simulink model "Roomba_Output_Cartesian"  (R2022b)
settings: Solver=FixedStepAuto  StartTime=0.0  StopTime=inf  FixedStep=0.02  RelTol=1e-3
undefined symbols (not defined in the file): b, offset_x, offset_y, theta_des, unicycle, X, x_des, x_f, Y, y_des, y_f
libraries: robotlib x3, dspsigops x1, simulink_extras x1
settings Model: Creator=Musta  LastModifiedBy=Musta
settings OptimizationCC: EnhancedBackFolding=on  PassReuseOutputArgsAs=Individual arguments  ZeroExternalMemoryAtStartup=off  ZeroInternalMemoryAtStartup=off  MaxStackSize=64  OptimizeBlockOrder=speed  DifferentSizesBufferReuse=on  OptimizationCustomize=off  EfficientTunableParamExpr=on
settings DebuggingCC: ParameterTunabilityLossMsg=error
settings HardwareCC: ProdBitPerPointer=32  ProdBitPerSizeT=32  ProdBitPerPtrDiffT=32  ProdLargestAtomicFloat=None  ProdIntDivRoundTo=Undefined  ProdEndianess=Unspecified  ProdWordSize=32  ProdHWDeviceType=Generic->Unspecified (assume 32-bit Generic)
settings SFSimCC: MATLABDynamicMemAlloc=off
settings RTWCC: Description=Embedded Coder  SystemTargetFile=ert.tlc  HardwareBoard=Robot Operating System (ROS)  TLCOptions="-aInlineSetEventsForThisBaseRateFcn=TLC_FALSE -aSuppressMultiTaskScheduler=TLC_FALSE  -aRateBasedStepFcn=0"  TemplateMakefile=ert_default_tmf  Toolchain=Catkin  TargetLang=C++
settings CodeAppCC: ForceParamTrailComments=on  IgnoreCustomStorageClasses=off  OperatorAnnotations=on  SimulinkDataObjDesc=on  SFDataObjDesc=on  InsertBlockDesc=on

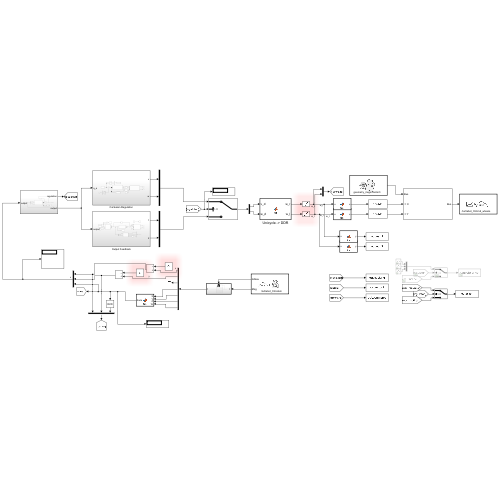
[thumbnail: Simulink's stored preview of the top-level diagram]
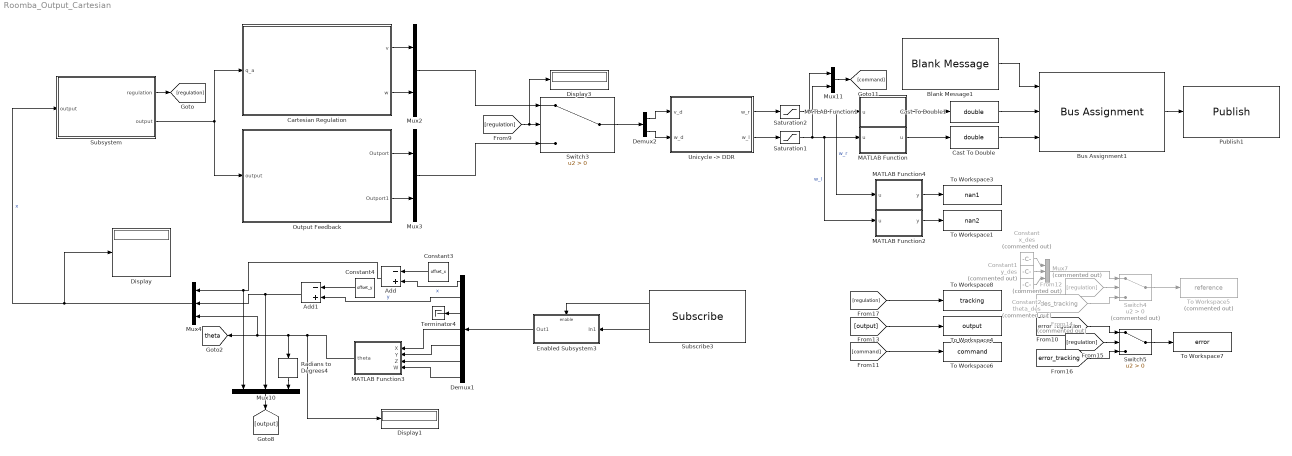
== system Roomba_Output_Cartesian ==
  Add : Sum  Inputs=-+
  Add1 : Sum  Inputs=-+
  Blank Message1 : robotlib/Blank Message  messageClass=Message  entityType=geometry_msgs/Vector3  messageType=geometry_msgs/Vector3  SampleTime=0.02  legacyBusStruct=off
      settings: LibrarySourceBlock=roslib/ROS/Blank Message
  Bus Assignment1 : BusAssignment  AssignedSignals=X,Y
  Cartesian Regulation : Subsystem
  Cast To Double : DataTypeConversion  OutDataTypeStr=double  SaturateOnIntegerOverflow=off  RndMeth=Floor
  Cast To Double1 : DataTypeConversion  OutDataTypeStr=double  SaturateOnIntegerOverflow=off  RndMeth=Floor
  Constant : Constant  Commented=on  Value=x_des
  Constant1 : Constant  Commented=on  Value=y_des
  Constant2 : Constant  Commented=on  Value=theta_des
  Constant3 : Constant  Value=offset_x
  Constant4 : Constant  Value=offset_y
  Demux1 : Demux  Outputs=7
  Demux2 : Demux  Outputs=2
  Display : Display
  Display1 : Display
  Display3 : Display
  Enabled Subsystem3 : Subsystem  TreatAsAtomicUnit=on
  From12 : From  Commented=on  GotoTag=regulation
  From14 : From  Commented=on  GotoTag=des_tracking  TagVisibility=global
  MATLAB Function : MATLAB Function  TreatAsAtomicUnit=on
  MATLAB Function1 : MATLAB Function  TreatAsAtomicUnit=on
  MATLAB Function2 : MATLAB Function  TreatAsAtomicUnit=on
  MATLAB Function3 : MATLAB Function  TreatAsAtomicUnit=on
  MATLAB Function4 : MATLAB Function  TreatAsAtomicUnit=on
  Mux10 : Mux  Inputs=3
  Mux11 : Mux  Inputs=2
  Mux2 : Mux  Inputs=2
  Mux3 : Mux  Inputs=2
  Mux4 : Mux  Inputs=3
  Mux7 : Mux  Commented=on  Inputs=3
  Output Feedback : Subsystem
  Publish1 : robotlib/Publish  topicSource=Select from ROS network  topic=/turtlebot_03/cmd_wheels  messageType=geometry_msgs/Vector3  legacyBusStruct=off  messageQueueLength=1
      settings: LibrarySourceBlock=roslib/ROS/Publish
  Radians to Degrees4 : simulink_extras/Transformations/Radians to Degrees
  Saturation1 : Saturate  UpperLimit=unicycle.omegaWheelMax  LowerLimit=unicycle.omegaWheelMin
  Saturation2 : Saturate  UpperLimit=unicycle.omegaWheelMax  LowerLimit=unicycle.omegaWheelMin
  Subscribe3 : robotlib/Subscribe  topicSource=Select from ROS network  topic=/turtlebot_03/odom  messageType=nav_msgs/Odometry  SampleTime=0.02  legacyBusStruct=off  messageQueueLength=1
      settings: LibrarySourceBlock=roslib/ROS/Subscribe
  Subsystem : Subsystem
  Switch3 : Switch  Criteria=u2 > Threshold  SaturateOnIntegerOverflow=off  InputSameDT=off
  Switch4 : Switch  Commented=on  Criteria=u2 > Threshold  SaturateOnIntegerOverflow=off  InputSameDT=off
  Switch5 : Switch  Criteria=u2 > Threshold  SaturateOnIntegerOverflow=off  InputSameDT=off
  Terminator4 : Terminator
  To Workspace1 : ToWorkspace  VariableName=nan2  SaveFormat=Structure With Time  SampleTime=-1
  To Workspace3 : ToWorkspace  VariableName=nan1  SaveFormat=Structure With Time  SampleTime=-1
  To Workspace4 : ToWorkspace  VariableName=output  SaveFormat=Structure With Time  SampleTime=-1
  To Workspace5 : ToWorkspace  Commented=on  VariableName=reference  SaveFormat=Structure With Time  SampleTime=-1
  To Workspace6 : ToWorkspace  VariableName=command  SaveFormat=Structure With Time  SampleTime=-1
  To Workspace7 : ToWorkspace  VariableName=error  SaveFormat=Structure With Time  SampleTime=-1
  To Workspace8 : ToWorkspace  VariableName=tracking  SaveFormat=Structure With Time  SampleTime=-1
  "Unicycle -> DDR" : MATLAB Function  TreatAsAtomicUnit=on
  tag scope: theta=global
  wires:
  Radians to Degrees4/1 -> Mux10/3
  "Unicycle -> DDR"/1(w_r) -> Saturation2/1
  MATLAB Function3/1(theta) -> Display1/1, Radians to Degrees4/1, Mux4/3, [theta]
  Subscribe3/2 -> Enabled Subsystem3/1(In1)
  Mux10/1 -> [output]
  Demux1/3 -> Terminator4/1
  Blank Message1/1 -> Bus Assignment1/1
  Bus Assignment1/1 -> Publish1/1
  Subscribe3/1 -> Enabled Subsystem3/Enable
  Mux11/1 -> [command]
  Enabled Subsystem3/1(Out1) -> Demux1/1
  From12/1 -> Switch4/2
  [regulation] -> To Workspace8/1
  Switch5/1 -> To Workspace7/1
  Constant1/1 -> Mux7/2
  Mux7/1 -> Switch4/1
  Demux2/2 -> "Unicycle -> DDR"/2(w_d)
  [output] -> To Workspace4/1
  [error_regulation] -> Switch5/1
  Constant/1 -> Mux7/1
  "Unicycle -> DDR"/2(w_l) -> Saturation1/1
  [regulation] -> Switch5/2
  From14/1 -> Switch4/3
  Switch4/1 -> To Workspace5/1
  Demux2/1 -> "Unicycle -> DDR"/1(v_d)
  [regulation] -> Display3/1, Switch3/2
  Mux2/1 -> Switch3/1
  [command] -> To Workspace6/1
  Switch3/1 -> Demux2/1
  [error_tracking] -> Switch5/3
  Mux3/1 -> Switch3/3
  Constant2/1 -> Mux7/3
  Mux4/1 -> Subsystem/1("output "), Display/1  "x"
  Demux1/1 -> Add/2  "x"
  Constant3/1 -> Add/1
  Constant4/1 -> Add1/1
  Demux1/2 -> Add1/2  "y"
  Add1/1 -> Mux4/2, Mux10/2
  Add/1 -> Mux4/1, Mux10/1
  Cast To Double1/1 -> Bus Assignment1/2
  Cast To Double/1 -> Bus Assignment1/3
  Output Feedback/2(Outport1) -> Mux3/2
  Output Feedback/1(Outport) -> Mux3/1
  Cartesian Regulation/1(v) -> Mux2/1
  Cartesian Regulation/2(w) -> Mux2/2
  Demux1/7 -> MATLAB Function3/4(W)
  Demux1/6 -> MATLAB Function3/3(Z)
  Demux1/4 -> MATLAB Function3/1(X)
  Demux1/5 -> MATLAB Function3/2(Y)
  Saturation1/1 -> MATLAB Function2/1(u), MATLAB Function/1("u "), Mux11/2  "w_l"
  Saturation2/1 -> MATLAB Function4/1(u), MATLAB Function1/1("u "), Mux11/1  "w_r"
  MATLAB Function/1(u) -> Cast To Double/1
  MATLAB Function2/1(y) -> To Workspace1/1
  MATLAB Function4/1(y) -> To Workspace3/1
  MATLAB Function1/1(u) -> Cast To Double1/1
  Subsystem/1(regulation) -> [regulation]
  Subsystem/2(output) -> Output Feedback/1(output), Cartesian Regulation/1(q_a)

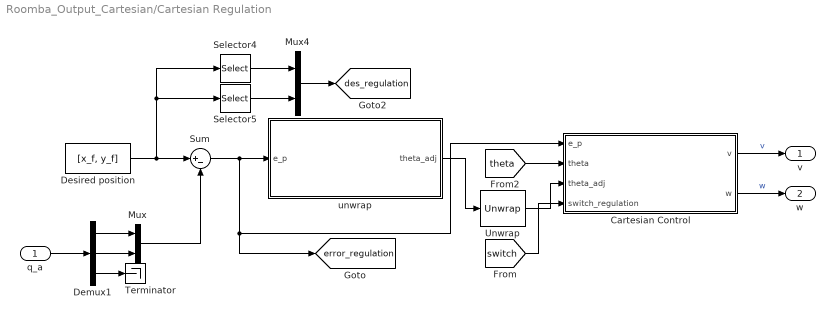
== system Roomba_Output_Cartesian/Cartesian Regulation ==
  q_a : Inport
  Cartesian Control : MATLAB Function  TreatAsAtomicUnit=on
  Demux1 : Demux  Outputs=3
  Desired position : Constant  Value=[x_f, y_f]
  Mux : Mux  Inputs=2
  Mux4 : Mux  Inputs=2
  Selector4 : Selector  InputPortWidth=2  IndexOptions=Index vector (dialog)  Indices=1  OutputSizes=1
  Selector5 : Selector  InputPortWidth=2  IndexOptions=Index vector (dialog)  Indices=2  OutputSizes=1
  Sum : Sum  Inputs=|+-
  Terminator : Terminator
  Unwrap : dspsigops/Unwrap  tol=0.99*pi  InputProcessing=Columns as channels (frame based)  running=off
  unwrap : MATLAB Function  TreatAsAtomicUnit=on
  v : Outport
  w : Outport  Port=2
  tag scope: des_regulation=global, error_regulation=global
  wires:
  Demux1/1 -> Mux/1
  Demux1/2 -> Mux/2
  q_a/1 -> Demux1/1
  unwrap/1(theta_adj) -> Unwrap/1
  Sum/1 -> [error_regulation], Cartesian Control/1(e_p), unwrap/1(e_p)
  Mux4/1 -> [des_regulation]
  Selector5/1 -> Mux4/2
  [theta] -> Cartesian Control/2(theta)
  Desired position/1 -> Selector4/1, Selector5/1, Sum/1
  Selector4/1 -> Mux4/1
  Unwrap/1 -> Cartesian Control/3(theta_adj)
  Mux/1 -> Sum/2
  Demux1/3 -> Terminator/1
  Cartesian Control/1(v) -> v/1  "v"
  Cartesian Control/2(w) -> w/1  "w"
  [switch] -> Cartesian Control/4(switch_regulation)

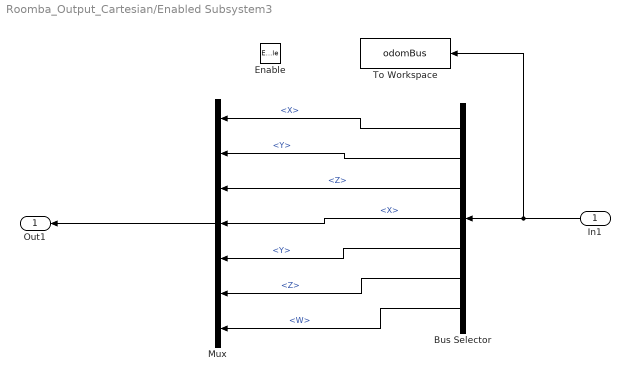
== system Roomba_Output_Cartesian/Enabled Subsystem3 ==
  In1 : Inport
  Enable : EnablePort
  Bus Selector : BusSelector  OutputSignals=Pose.Pose.Position.X,Pose.Pose.Position.Y,Pose.Pose.Position.Z,Pose.Pose.Orientation.X,Pose.Pose.Orientation.Y,Pose.Pose.Orientation.Z,Pose.Pose.Orientation.W
  Mux : Mux  Inputs=7
  To Workspace : ToWorkspace  VariableName=odomBus  SaveFormat=Timeseries  SampleTime=-1
  Out1 : Outport
  wires:
  Mux/1 -> Out1/1
  Bus Selector/1 -> Mux/1  "<X>"
  Bus Selector/2 -> Mux/2  "<Y>"
  In1/1 -> To Workspace/1, Bus Selector/1
  Bus Selector/3 -> Mux/3  "<Z>"
  Bus Selector/4 -> Mux/4  "<X>"
  Bus Selector/5 -> Mux/5  "<Y>"
  Bus Selector/6 -> Mux/6  "<Z>"
  Bus Selector/7 -> Mux/7  "<W>"

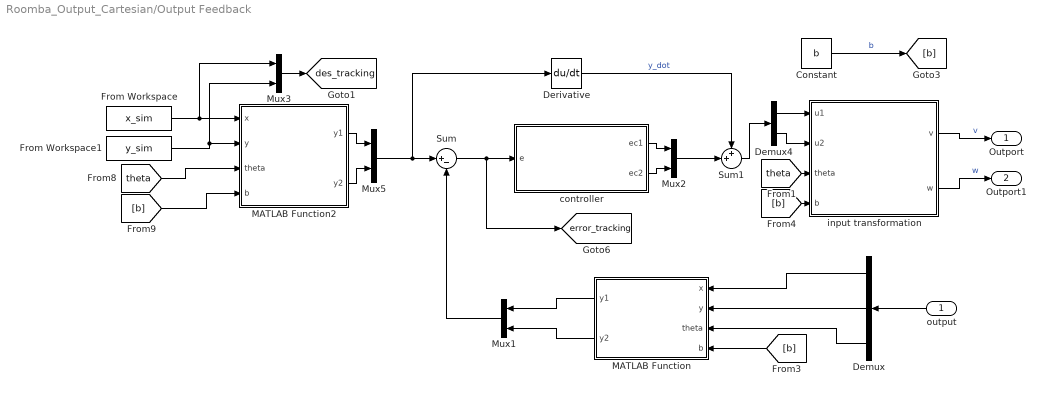
== system Roomba_Output_Cartesian/Output Feedback ==
  output : Inport
  Constant : Constant  Value=b
  Demux : Demux  Outputs=3
  Demux4 : Demux  Outputs=2
  Derivative : Derivative
  From Workspace : FromWorkspace  VariableName=x_sim
  From Workspace1 : FromWorkspace  VariableName=y_sim
  MATLAB Function : MATLAB Function  TreatAsAtomicUnit=on
  MATLAB Function2 : MATLAB Function  TreatAsAtomicUnit=on
  Mux{1..3,5} (4 alike) : Mux  Inputs=2
  Sum : Sum  Inputs=|+-
  Sum1 : Sum  Inputs=++|
  controller : MATLAB Function  TreatAsAtomicUnit=on
  input transformation : MATLAB Function  TreatAsAtomicUnit=on
  Outport : Outport
  Outport1 : Outport  Port=2
  tag scope: des_tracking=global, error_tracking=global
  wires:
  controller/1(ec1) -> Mux2/1
  Mux5/1 -> Derivative/1, Sum/1
  MATLAB Function2/2(y2) -> Mux5/2
  Mux3/1 -> [des_tracking]
  [b] -> MATLAB Function2/4(b)
  Derivative/1 -> Sum1/1  "y_dot"
  [b] -> input transformation/4(b)
  Demux4/2 -> input transformation/2(u2)
  Demux4/1 -> input transformation/1(u1)
  [theta] -> MATLAB Function2/3(theta)
  Sum/1 -> [error_tracking], controller/1(e)
  From Workspace1/1 -> Mux3/2, MATLAB Function2/2(y)
  Mux1/1 -> Sum/2
  MATLAB Function/2(y2) -> Mux1/2
  [b] -> MATLAB Function/4(b)
  [theta] -> input transformation/3(theta)
  input transformation/2(w) -> Outport1/1  "w"
  MATLAB Function2/1(y1) -> Mux5/1
  Sum1/1 -> Demux4/1
  controller/2(ec2) -> Mux2/2
  input transformation/1(v) -> Outport/1  "v"
  Constant/1 -> [b]  "b"
  From Workspace/1 -> Mux3/1, MATLAB Function2/1(x)
  MATLAB Function/1(y1) -> Mux1/1
  Mux2/1 -> Sum1/2
  output/1 -> Demux/1
  Demux/1 -> MATLAB Function/1(x)
  Demux/2 -> MATLAB Function/2(y)
  Demux/3 -> MATLAB Function/3(theta)

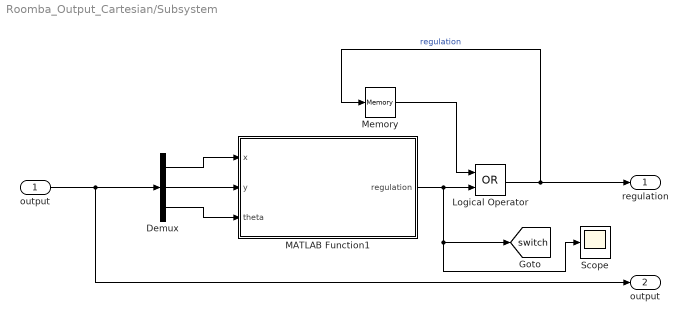
== system Roomba_Output_Cartesian/Subsystem ==
  "output " : Inport
  Demux : Demux  Outputs=3
  Logical Operator : Logic  Operator=OR  AllPortsSameDT=off  OutDataTypeStr=boolean
  MATLAB Function1 : MATLAB Function  TreatAsAtomicUnit=on
  Memory : Memory
  Scope : Scope
  regulation : Outport
  output : Outport  Port=2
  tag scope: switch=global
  wires:
  Memory/1 -> Logical Operator/1
  Logical Operator/1 -> regulation/1, Memory/1  "regulation"
  MATLAB Function1/1(regulation) -> [switch], Scope/1, Logical Operator/2
  "output "/1 -> output/1, Demux/1
  Demux/3 -> MATLAB Function1/3(theta)
  Demux/2 -> MATLAB Function1/2(y)
  Demux/1 -> MATLAB Function1/1(x)

== matlab function Roomba_Output_Cartesian/Cartesian Regulation/unwrap ==
  data: theta_adj output; e_p input

function theta_adj = unwrap(e_p)

    theta_adj = mod(atan2(e_p(2),e_p(1)),2*pi);

end

== matlab function Roomba_Output_Cartesian/Subsystem/MATLAB Function1 ==
  data: x input; regulation output; y input; theta input
function regulation = fcn(x,y,theta)

    y_des = 1.51;
    x_des = -0.5;

    th = 0.01;

    if (abs(x)<abs(x_des)+th) && (abs(x)>abs(x_des)-th) && (abs(y)<abs(y_des)+th) && (abs(y)>abs(y_des)-th)
        regulation = 1;
    else
        regulation = 0;
    end

end

== matlab function Roomba_Output_Cartesian/Unicycle -> DDR ==
  data: v_d input; w_r output; w_d input; w_l output
function [w_r, w_l] = fcn(v_d, w_d)

    d = 0.165;
    r = 0.034;

    w_r = ((2 * v_d) + (w_d * d)) / (2 * r);
    w_l = ((2 * v_d) - (w_d * d)) / (2 * r);

end

== matlab function Roomba_Output_Cartesian/Output Feedback/MATLAB Function ==
  data: x input; y1 output; y input; theta input; b input; y2 output
function [y1,y2] = p2y(x,y,theta,b)

    y1 = x + b*cos(theta);
    y2 = y + b*sin(theta);
    
end

== matlab function Roomba_Output_Cartesian/MATLAB Function3 ==
  data: X input; theta output; Y input; Z input; W input
function theta = fcn(X, Y, Z, W)

    theta = 2*acos(W);
    
end

== matlab function Roomba_Output_Cartesian/MATLAB Function ==
  data: u input; u output
function u = fcn(u)


    if (isnan(u))
        u = 0.1;
    end

end

== matlab function Roomba_Output_Cartesian/MATLAB Function1 ==
  data: u input; u output
function u = fcn(u)

    if (isnan(u))
        u = 0.1;
    end

end

== matlab function Roomba_Output_Cartesian/Output Feedback/MATLAB Function2 ==
  data: x input; y1 output; y input; y2 output; theta input; b input
function [y1,y2] = p2y(x,y,theta,b)

y1 = x + b*cos(theta);
y2 = y + b*sin(theta);

== matlab function Roomba_Output_Cartesian/MATLAB Function2 ==
  data: u input; y output
function y = fcn(u)

    y = 0;

    if (isnan(u))
        y = 1;
    end

end

== matlab function Roomba_Output_Cartesian/Output Feedback/controller ==
  data: e input; ec1 output; ec2 output
function [ec1, ec2] = fcn(e)

    %#codegen
    coder.extrinsic('evalin')
    k1 = 0;                  % Needed in order to set variable class correctly
    k2 = 0;                  % Needed in order to set variable class correctly
    k1 = evalin('base','k1'); % Read value from workspace
    k2 = evalin('base','k2'); % Read value from workspace
    
    ec1 = k1*(e(1));
    ec2 = k2*(e(2));
    
end

== matlab function Roomba_Output_Cartesian/MATLAB Function4 ==
  data: u input; y output
function y = fcn(u)

    y = 0;

    if (isnan(u))
        y = 1;
    end

end

== matlab function Roomba_Output_Cartesian/Output Feedback/input transformation ==
  data: u1 input; u2 input; theta input; v output; b input; w output
function [v,w] = fcn(u1, u2, theta, b)

    R = [cos(theta),      sin(theta);
         -sin(theta)/b, cos(theta)/b];
    
    v = cos(theta)*u1 + sin(theta)*u2;
    w = (-sin(theta)/b)*u1 + (cos(theta)/b)*u2;

end

== matlab function Roomba_Output_Cartesian/Cartesian Regulation/Cartesian Control ==
  data: v output; w output; e_p input; theta input; theta_adj input; switch_regulation input
function [v,w] = cartesian_controller(e_p, theta, theta_adj, switch_regulation)

    %#codegen
    coder.extrinsic('evalin')
    K_v = 0;                  % Needed in order to set variable class correctly
    K_w = 0;                  % Needed in order to set variable class correctly
    K_v = evalin('base','K_v'); % Read value from workspace
    K_w = evalin('base','K_w'); % Read value from workspace

    if switch_regulation
        if theta<0
            theta = theta+2*pi;
        end
    end

    v = K_v * (e_p(1)*cos(theta) + e_p(2)*sin(theta));
    w = K_w * (theta_adj - theta);

end
